simulink model "verify_Absorption_Chiller_LookUp_mdl"  (R2018b)
settings: Solver=ode45  StartTime=0.0  StopTime=3600  MaxStep=60  RelTol=1e-3  EnableMultiTasking=on
libraries: carnot x4
settings Model: Creator=drhf  LastModifiedBy=drhf
settings DataIOCC: SaveFormat=Array  SignalLogging=off  DSMLogging=off
settings OptimizationCC: ExpressionDepthLimit=2147483647  LifeSpan=inf
settings DebuggingCC: SolverPrmCheckMsg=warning  StateNameClashWarn=warning  SFUnexpectedBacktrackingDiag=warning  SFNoUnconditionalDefaultTransitionDiag=warning  SFExecutionAtInitializationDiag=none
settings HardwareCC: ProdBitPerPointer=32  ProdBitPerSizeT=32  ProdBitPerPtrDiffT=32  ProdLargestAtomicFloat=None  ProdIntDivRoundTo=Undefined  ProdEndianess=Unspecified  ProdWordSize=32  ProdHWDeviceType=32-bit Generic
settings ModelReferenceCC: PropagateSignalLabelsOutOfModel=off
settings SFSimCC: SimUseLocalCustomCode=off
settings RTWCC: RTWUseLocalCustomCode=off
settings CodeAppCC: StateflowObjectComments=on
settings GRTTargetCC: TargetLangStandard=C89/C90 (ANSI)  GeneratePreprocessorConditionals=Disable all  CombineOutputUpdateFcns=off  GRTInterface=on
settings ConfigComp: CovMetricSettings=dw  CovHtmlReporting=on  CovSaveCumulativeToWorkspaceVar=on  CovSaveSingleToWorkspaceVar=on  CovExternalEMLEnable=off

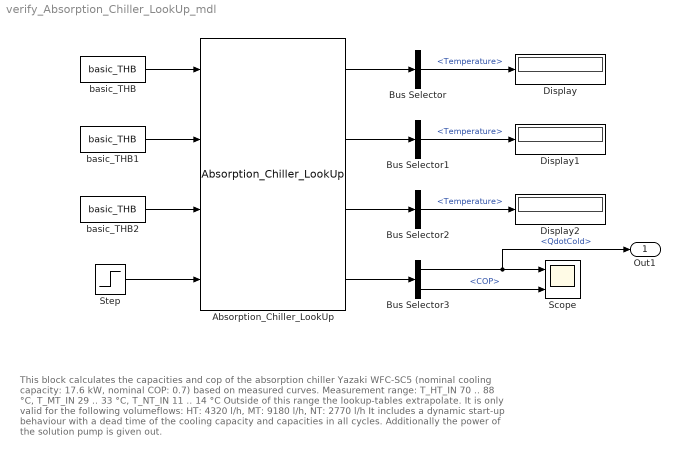
== system verify_Absorption_Chiller_LookUp_mdl ==
  note: This block calculates the capacities and cop of the absorption chiller Yazaki WFC-SC5 (nominal cooling capacity: 17.6 kW, nominal COP: 0.7) based on measured curves.
      | Measurement range:
      | T_HT_IN 70 .. 88 °C, T_MT_IN 29 .. 33 °C, T_NT_IN 11 .. 14 °C
      | Outside of this range the lookup-tables extrapolate.
      |
      | It is only valid for the following volumeflows:
      | HT: 4320 l/h, MT: 9180 l/h, NT: 2770 l/h
      |
      | It includes a dynamic start-up behaviour with a dead time of the cooling capacity and capacities in all cycles.
      | Additionally the power of the solution pump is given out.
  Absorption_Chiller_LookUp : carnot/Source/Chiller/Absorption_Chiller_LookUp  chillertype=Yazaki WFC-SC5  heating_T_heating=[70 71 72 73 74 75 76 77 78 79 80 81 82 83 84 85 86 87 88]  heating_T_recooling=[29 31 33]  heating_T_cooling=[11 12.5 14]  heating_Qdot=1000*cat(3, [11.5881 9.1729 7.1257; 12.7010 10.3602 8.4661; 13.7629 11.4453 9.5786; 14.7846 12.4541 10.5382; 15.7779 13.4104 11.3994; 16.7568 14.3365 12.1994; 17.7369 15.2538 12.9661; 18.7352 16.1871 13.7316; 19.7725 17.1783 14.5620; 20.8727 18.2790 15.5386; 21.4613 18.7997 16.0051; 22.1221 19.4526 16.6571; 22.8301 20.1885 17.4171; 23.5620 20.9610 18.2116; 24.3132 21.7625 19.0310; 25.0838 22.5963 19.8849; 25.8734 23.4650 20.7822; 26.6798 24.3672 21.7227; 27.5000 25.3000 22.7026], [11.5770 9.1404 7.0019; 12.7946 10.4820 8.5464; 13.9519 11.6809 9.7954; 15.0589 12.7736 10.8503; 16.1256 13.7910 11.7810; 17.1622 14.7571 12.6313; 18.1791 15.6924 13.4319; 19.1897 16.6217 14.2164; 20.2208 17.5967 15.0560; 21.3053 18.6810 16.0354; 21.9686 19.2406 16.5703; 22.7017 19.9403 17.2856; 23.4728 20.7187 18.0972; 24.2533 21.5195 18.9268; 25.0400 22.3359 19.7666; 25.8372 23.1759 20.6298; 26.6482 24.0459 21.5289; 27.4705 24.9436 22.4620; 28.3000 25.8635 23.4225], [11.6060 9.2707 7.0732; 12.8444 10.5919 8.6463; 14.0314 11.8008 9.9499; 15.1740 12.9258 11.0711; 16.2788 13.9911 12.0715; 17.3504 15.0094 12.9866; 18.3927 15.9884 13.8393; 19.4114 16.9403 14.6560; 20.4215 17.9043 15.5008; 21.4421 18.9298 16.4494; 22.3770 19.7105 17.1376; 23.3307 20.5777 17.9644; 24.2859 21.4864 18.8566; 25.2275 22.3953 19.7465; 26.1572 23.3020 20.6298; 27.0823 24.2153 21.5215; 28.0081 25.1426 22.4350; 28.9326 26.0813 23.3675; 29.8510 27.0252 24.3106])  recooling_T_heating=[70 79 88]  recooling_T_recooling=[29 31 33]  recooling_T_cooling=[11 12.5 14]  recooling_Qdot=1000*cat(3, [17.7490 12.9282 8.7004; 34.7262 30.2580 25.0504; 45.9087 40.8416 35.7528], [17.2271 12.0716 8.2439; 35.4258 31.2730 26.0419; 48.6320 43.2955 38.4385], [17.2978 12.4414 8.1943; 35.0711 30.8160 26.3417; 52.3435 45.8810 40.5337])  cooling_T_heating=[70 79 88]  cooling_T_recooling=[29 31 33]  cooling_T_cooling=[11 12.5 14]  cooling_Qdot=1000*cat(3, [7.0144 4.7740 2.6867; 14.9294 12.8469 10.4033; 19.0103 16.2646 13.7101], [6.8604 4.4520 2.5150; 15.2614 13.2863 10.9945; 20.4077 17.6879 15.3832], [6.9061 4.7080 2.6441; 15.1135 13.2179 11.1459; 22.6100 19.5272 17.0154])  deadtime_factor=11768  deadtime_exponent=-1.205
      settings: AttributesFormatString=%<chillertype>
  Bus Selector : BusSelector  OutputSignals=Temperature
  Bus Selector1 : BusSelector  OutputSignals=Temperature
  Bus Selector2 : BusSelector  OutputSignals=Temperature
  Bus Selector3 : BusSelector  OutputSignals=QdotCold,COP
  Display : Display
  Display1 : Display
  Display2 : Display
  Scope : Scope  NumInputPorts=2
  Step : Step  Time=600  SampleTime=0
  basic_THB : carnot/Basic/Hydraulics/basic_THB  t=88  mdot=4320/3600  p=1e5  ID=Pressure Drop from Massflow  fluid=Water  mix=0  mix2=0  mix3=0  dia=0.02  hgt=0
  basic_THB1 : carnot/Basic/Hydraulics/basic_THB  t=12.5  mdot=2770/3600  p=1e5  ID=Pressure Drop from Massflow  fluid=Water  mix=0  mix2=0  mix3=0  dia=0.02  hgt=0
  basic_THB2 : carnot/Basic/Hydraulics/basic_THB  t=31  mdot=9180/3600  p=1e5  ID=Pressure Drop from Massflow  fluid=Water  mix=0  mix2=0  mix3=0  dia=0.02  hgt=0
  Out1 : Outport
  wires:
  basic_THB/1 -> Absorption_Chiller_LookUp/1
  basic_THB1/1 -> Absorption_Chiller_LookUp/2
  basic_THB2/1 -> Absorption_Chiller_LookUp/3
  Step/1 -> Absorption_Chiller_LookUp/4
  Absorption_Chiller_LookUp/1 -> Bus Selector/1
  Bus Selector/1 -> Display/1  "<Temperature>"
  Absorption_Chiller_LookUp/2 -> Bus Selector1/1
  Bus Selector1/1 -> Display1/1  "<Temperature>"
  Bus Selector2/1 -> Display2/1  "<Temperature>"
  Absorption_Chiller_LookUp/3 -> Bus Selector2/1
  Absorption_Chiller_LookUp/4 -> Bus Selector3/1
  Bus Selector3/1 -> Out1/1, Scope/1  "<QdotCold>"
  Bus Selector3/2 -> Scope/2  "<COP>"
